simulink model "PI_TEST"  (R2020b)
settings: Solver=VariableStepAuto  StartTime=0.0  StopTime=6.283  RelTol=1e-3
libraries: simulink x1
settings Model: Creator=YUXIN  LastModifiedBy=YUXIN

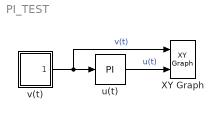
== system PI_TEST ==
  XY Graph : simulink/Sinks/XY Graph  xmin=-4  xmax=6  ymin=-15  ymax=15  st=0.001
  u(t) : S-Function  FunctionName=PI  SFunctionModules='PI'  SFunctionDeploymentMode=off  EnableBusSupport=off
  v(t) : Subsystem
      mask Display: disp('v(t)')
  wires:
  u(t)/1 -> XY Graph/2  "u(t)"
  v(t)/1(Out1) -> XY Graph/1, u(t)/1  "v(t)"

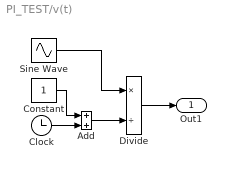
== system PI_TEST/v(t) ==
  Add : Sum
  Clock : Clock
  Constant : Constant
  Divide : Product  Inputs=*/
  Sine Wave : Sin  Amplitude=8  Frequency=3  SampleTime=0
  Out1 : Outport
  wires:
  Clock/1 -> Add/2
  Constant/1 -> Add/1
  Sine Wave/1 -> Divide/1
  Add/1 -> Divide/2
  Divide/1 -> Out1/1
